simulink model "Neutral_current_Load_balancing"  (R2019b)
settings: Solver=ode3  StartTime=0.0  StopTime=1  FixedStep=1e-6  MaxStep=1e-5  RelTol=1e-3
libraries: powerlib x39, powerlib_meascontrol x12, simulink x3, dsparch4 x1, eeHysteresisControl x1
settings Model: Creator=ASUS  LastModifiedBy=ASUS

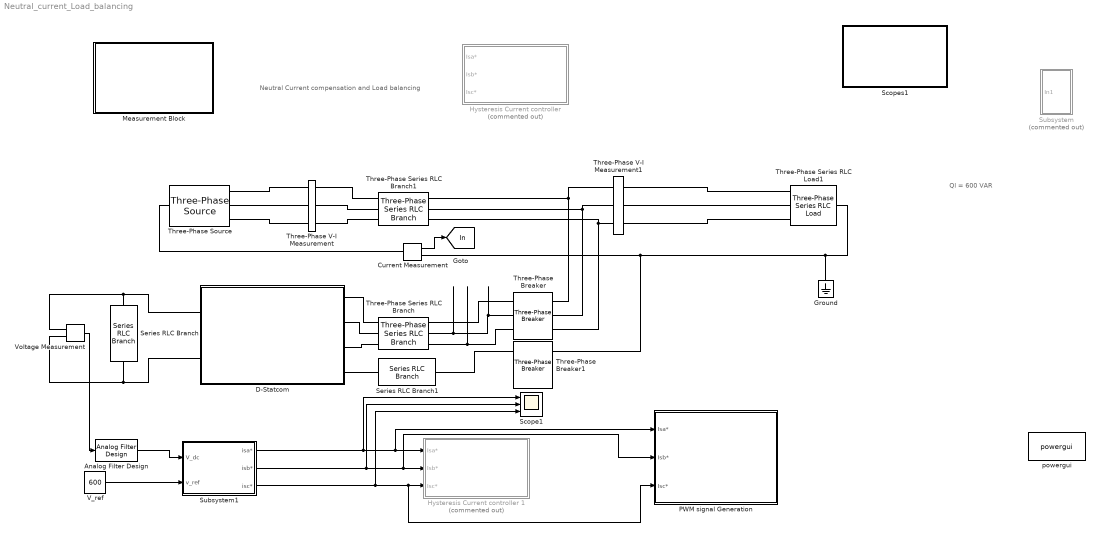
== system Neutral_current_Load_balancing ==
  note: Neutral Current compensation and Load balancing
  note: Ql = 600 VAR
  Analog Filter Design : dsparch4/Analog Filter Design  method=Butterworth  filttype=Lowpass  N=8  Wlo=75*2*pi  Whi=80  Rp=2  Rs=40
  Current Measurement : powerlib/Measurements/Current Measurement  PhasorSimulation=off  OutputType=Complex  PSBequivalent=0
      settings: SourceProductName=Simscape Electrical
  "D-Statcom " : Subsystem
  Ground : powerlib/Elements/Ground  LConnTagsString=a
      settings: SourceProductName=Simscape Electrical
  "Hysteresis Current controller " : Subsystem  Commented=on
  Hysteresis Current controller 1 : Subsystem  Commented=on
  Measurement Block : Subsystem
  PWM signal Generation : Subsystem
  Scope1 : Scope  NumInputPorts=3
  Scopes1 : Subsystem
  Series RLC Branch : powerlib/Elements/Series RLC Branch  LConnTagsString=__new0  RConnTagsString=__new0  BranchType=C  Resistance=1  Inductance=1e-3  SetiL0=off  InitialCurrent=0  Capacitance=10000e-6  Setx0=on  InitialVoltage=600  Measurements=None
      settings: SourceProductName=Simscape Electrical
  Series RLC Branch1 : powerlib/Elements/Series RLC Branch  LConnTagsString=__new0  RConnTagsString=__new0  BranchType=RL  Resistance=0.01  Inductance=12e-3  SetiL0=off  InitialCurrent=0  Capacitance=1e-6  Setx0=off  InitialVoltage=0  Measurements=None
      settings: SourceProductName=Simscape Electrical
  Subsystem : Subsystem  Commented=on
  Subsystem1 : Subsystem
  Three-Phase Series RLC Branch : powerlib/Elements/Three-Phase Series RLC Branch  LConnTagsString=A|B|C  RConnTagsString=A|B|C  BranchType=RL  Resistance=0.01  Inductance=10e-3  Capacitance=1e-6  Measurements=None
      settings: SourceProductName=Simscape Electrical
  Three-Phase Series RLC Branch1 : powerlib/Elements/Three-Phase Series RLC Branch  LConnTagsString=A|B|C  RConnTagsString=A|B|C  BranchType=RL  Resistance=0.01  Inductance=3.35e-3  Capacitance=1e-6  Measurements=None
      settings: SourceProductName=Simscape Electrical
  Three-Phase Series RLC Load1 : powerlib/Elements/Three-Phase Series RLC Load  LConnTagsString=A|B|C  RConnTagsString=N  Configuration=Y (neutral)  NominalVoltage=sqrt(6)*100  Vabc=[100 100 100]  Vabcp=[1e3 1e3 1e3]  NominalFrequency=50  UnbalancedPower=on  ActivePower=800  InductivePower=1000  CapacitivePower=0  Pabc=[100 200 300]  QLabc=[200 150 300]  QCabc=[0 0 0]  Pabcp=[10e3 9e3 11e3]  QLabcp=[100 90 110]  QCabcp=[100 90 110]  Measurements=None  LoadType=constant Z
      settings: SourceProductName=Simscape Electrical
  Three-Phase V-I Measurement : powerlib/Measurements/Three-Phase V-I Measurement  VoltageMeasurement=phase-to-ground  SetLabelV=on  LabelV=Vs  Vpu=off  VpuLL=off  CurrentMeasurement=yes  SetLabelI=on  LabelI=Is  Ipu=off  Pbase=100e6  Vbase=500e3  OutputType=Complex  PhasorSimulation=off  PSBequivalent=0
      settings: SourceProductName=Simscape Electrical
  Three-Phase V-I Measurement1 : powerlib/Measurements/Three-Phase V-I Measurement  VoltageMeasurement=phase-to-ground  SetLabelV=on  LabelV=Vr  Vpu=off  VpuLL=off  CurrentMeasurement=yes  SetLabelI=on  LabelI=Ir  Ipu=off  Pbase=100e6  Vbase=500e3  OutputType=Complex  PhasorSimulation=off  PSBequivalent=0
      settings: SourceProductName=Simscape Electrical
  Three-Phase Breaker : powerlib/Elements/Three-Phase Breaker  InitialState=open  SwitchA=on  SwitchB=on  SwitchC=on  SwitchTimes=[0.1 0.6]  External=off  BreakerResistance=0.01  SnubberResistance=1e6  SnubberCapacitance=inf  Measurements=None
      settings: SourceProductName=Simscape Electrical
  Three-Phase Breaker1 : powerlib/Elements/Three-Phase Breaker  InitialState=open  SwitchA=on  SwitchB=off  SwitchC=off  SwitchTimes=[0.1 0.6]  External=off  BreakerResistance=0.01  SnubberResistance=1e6  SnubberCapacitance=inf  Measurements=None
      settings: SourceProductName=Simscape Electrical
  Three-Phase Source : powerlib/Electrical Sources/Three-Phase Source  InternalConnection=Yn  VoltagePhases=off  Voltage=100*sqrt(6)  PhaseAngle=0  Voltage_phases=[25e3 25e3 25e3]/sqrt(3)  PhaseAngles_phases=[0 -120 +120]  Frequency=50  NonIdealSource=off  SpecifyImpedance=off  Resistance=0.8929  Inductance=16.58e-3  ShortCircuitLevel=100e6  BaseVoltage=sqrt(2)*100  XRratio=7  BusType=swing  Pref=10e3  Qref=0  Prefabc=[10e3, 10e3, 10e3]  Qrefabc=[0, 0, 0]  Qmin=-inf  Qmax=inf
      settings: SourceProductName=Simscape Electrical
  V_ref : Constant  Value=600
  Voltage Measurement : powerlib/Measurements/Voltage Measurement  PhasorSimulation=off  OutputType=Complex  PSBequivalent=0
      settings: SourceProductName=Simscape Electrical
  powergui : powerlib/powergui  Priority=1  SimulationMode=Discrete  SampleTime=1e-6  frequency=60  Iterations=50  frequencyindice=50  Pbase=100e6  ErrMax=1e-4  UnitsV=kV  UnitsW=MW  buscounter=0  FunctionMessages=off  echomessages=off  EnableUseOfTLC=off  CurrentSourceSwitches=off  DisableSnubberDevices=off  DisableRonSwitches=off  DisableVfSwitches=off  DisplayEquations=off  AutomaticDiscreteSolvers=off  SolverType=Tustin/Backward Euler (TBE)  Interpol=off  ExternalGateDelay=off  methode=off  Ts=100  x0status=blocks  SPID=on  SwTol=0  HookPort=off  NonlinearTolerance=1e-4  nMaxIteration=100  ContinueOnMaxIteration=off  RestoreLinks=warning  ResistiveCurrentMeasurement=off  Frange=[0:2:500]  Ylog=off  Xlog=on  ShowGrid=off  save=off  variable=ZData  structure=0  ZoomFFT=off  StartTime=0.0  cycles=1  DisplayStyle=1  fundamental=60  FreqAxis=off  MaxFrequency=1000  frequencyindicesteady=1  RmsSteady=1  display=off
      settings: SourceProductName=Simscape Electrical
  tag scope: In=global
  wires:
  Subsystem1/1(isa*) -> PWM signal Generation/1(Isa*), Hysteresis Current controller 1/1(Isa*), Scope1/1
  Subsystem1/2(isb*) -> PWM signal Generation/2(Isb*), Hysteresis Current controller 1/2(Isb*), Scope1/2
  Subsystem1/3(isc*) -> PWM signal Generation/3(Isc*), Hysteresis Current controller 1/3(Isc*), Scope1/3
  V_ref/1 -> Subsystem1/2(v_ref)
  Voltage Measurement/1 -> Analog Filter Design/1
  Analog Filter Design/1 -> Subsystem1/1(V_dc)
  Current Measurement/1 -> [In]
  connections:
  Three-Phase Series RLC Branch/LConn1 -- "D-Statcom "/RConn1
  "D-Statcom "/RConn2 -- Three-Phase Series RLC Branch/LConn2
  "D-Statcom "/RConn3 -- Three-Phase Series RLC Branch/LConn3
  "D-Statcom "/LConn1 -- Voltage Measurement/LConn1 -- Series RLC Branch/LConn1
  "D-Statcom "/LConn2 -- Series RLC Branch/RConn1 -- Voltage Measurement/LConn2
  Three-Phase V-I Measurement/LConn1 -- Three-Phase Source/RConn1
  Three-Phase Source/RConn2 -- Three-Phase V-I Measurement/LConn2
  Three-Phase Source/RConn3 -- Three-Phase V-I Measurement/LConn3
  Three-Phase Breaker/RConn1 -- Three-Phase V-I Measurement1/LConn1 -- Three-Phase Series RLC Branch1/RConn1
  Three-Phase Breaker/RConn2 -- Three-Phase V-I Measurement1/LConn2 -- Three-Phase Series RLC Branch1/RConn2
  Three-Phase Breaker/RConn3 -- Three-Phase Series RLC Branch1/RConn3 -- Three-Phase V-I Measurement1/LConn3
  Three-Phase Series RLC Load1/LConn1 -- Three-Phase V-I Measurement1/RConn1
  Three-Phase Series RLC Load1/LConn2 -- Three-Phase V-I Measurement1/RConn2
  Three-Phase Series RLC Load1/LConn3 -- Three-Phase V-I Measurement1/RConn3
  Three-Phase Breaker/LConn1 -- Three-Phase Series RLC Branch/RConn1
  Three-Phase Breaker/LConn2 -- Three-Phase Series RLC Branch/RConn2
  Three-Phase Breaker/LConn3 -- Three-Phase Series RLC Branch/RConn3
  Three-Phase Series RLC Branch1/LConn1 -- Three-Phase V-I Measurement/RConn1
  Three-Phase V-I Measurement/RConn2 -- Three-Phase Series RLC Branch1/LConn2
  Three-Phase Series RLC Branch1/LConn3 -- Three-Phase V-I Measurement/RConn3
  Series RLC Branch1/LConn1 -- "D-Statcom "/RConn4
  Current Measurement/RConn1 -- Three-Phase Breaker1/RConn1 -- Ground/LConn1 -- Three-Phase Series RLC Load1/RConn1
  Series RLC Branch1/RConn1 -- Three-Phase Breaker1/LConn1
  Current Measurement/LConn1 -- Three-Phase Source/LConn1

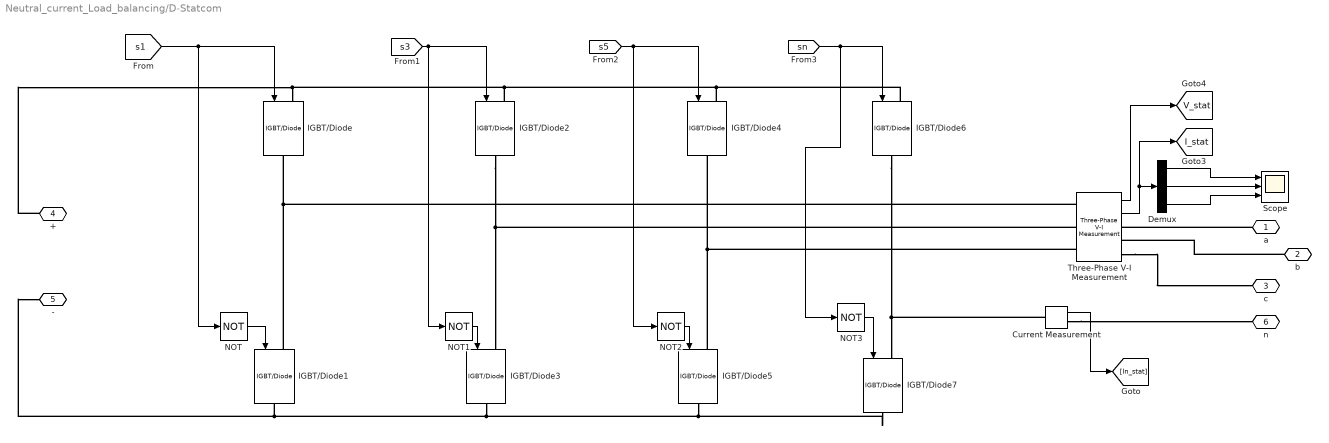
== system Neutral_current_Load_balancing/D-Statcom  ==
  Current Measurement : powerlib/Measurements/Current Measurement  PhasorSimulation=off  OutputType=Complex  PSBequivalent=0
      settings: SourceProductName=Simscape Electrical
  Demux : Demux  Outputs=3
  IGBT/Diode{,1..7} (8 alike) : powerlib/Power Electronics/IGBT//Diode  Ron=1e-3  Rs=1e5  Cs=inf  Measurements=off
      settings: SourceProductName=Simscape Electrical
  NOT{,1..3} (4 alike) : Logic  Operator=NOT  IconShape=distinctive  AllPortsSameDT=off  OutDataTypeStr=boolean
  Scope : Scope  NumInputPorts=3
  Three-Phase V-I Measurement : powerlib/Measurements/Three-Phase V-I Measurement  VoltageMeasurement=phase-to-ground  SetLabelV=off  LabelV=Vabc  Vpu=off  VpuLL=off  CurrentMeasurement=yes  SetLabelI=off  LabelI=Iabc  Ipu=off  Pbase=100e6  Vbase=500e3  OutputType=Complex  PhasorSimulation=off  PSBequivalent=0
      settings: SourceProductName=Simscape Electrical
  a : PMIOPort  Side=Right
  b : PMIOPort  Port=2  Side=Right
  c : PMIOPort  Port=3  Side=Right
  + : PMIOPort  Port=4  Side=Left
  - : PMIOPort  Port=5  Side=Left
  n : PMIOPort  Port=6  Side=Right
  tag scope: I_stat=global, V_stat=global
  wires:
  [s1] -> NOT/1, IGBT/Diode/1
  [s5] -> NOT2/1, IGBT/Diode4/1
  NOT2/1 -> IGBT/Diode5/1
  NOT/1 -> IGBT/Diode1/1
  [s3] -> IGBT/Diode2/1, NOT1/1
  NOT1/1 -> IGBT/Diode3/1
  Three-Phase V-I Measurement/2 -> [I_stat], Demux/1
  Demux/1 -> Scope/1
  Demux/2 -> Scope/2
  Demux/3 -> Scope/3
  Three-Phase V-I Measurement/1 -> [V_stat]
  [sn] -> NOT3/1, IGBT/Diode6/1
  NOT3/1 -> IGBT/Diode7/1
  Current Measurement/1 -> [In_stat]
  connections:
  IGBT/Diode1/RConn1 -- -/RConn1 -- IGBT/Diode7/RConn1 -- IGBT/Diode5/RConn1 -- IGBT/Diode3/RConn1
  IGBT/Diode2/LConn1 -- IGBT/Diode6/LConn1 -- IGBT/Diode4/LConn1 -- +/RConn1 -- IGBT/Diode/LConn1
  IGBT/Diode1/LConn1 -- Three-Phase V-I Measurement/LConn1 -- IGBT/Diode/RConn1
  IGBT/Diode2/RConn1 -- IGBT/Diode3/LConn1 -- Three-Phase V-I Measurement/LConn2
  IGBT/Diode5/LConn1 -- Three-Phase V-I Measurement/LConn3 -- IGBT/Diode4/RConn1
  a/RConn1 -- Three-Phase V-I Measurement/RConn1
  b/RConn1 -- Three-Phase V-I Measurement/RConn2
  Three-Phase V-I Measurement/RConn3 -- c/RConn1
  IGBT/Diode6/RConn1 -- Current Measurement/LConn1 -- IGBT/Diode7/LConn1
  Current Measurement/RConn1 -- n/RConn1

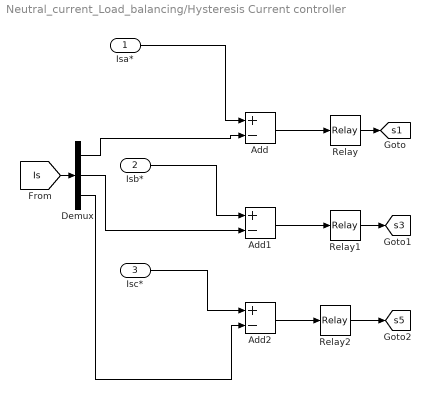
== system Neutral_current_Load_balancing/Hysteresis Current controller  ==
  Isa* : Inport
  Isb* : Inport  Port=2
  Isc* : Inport  Port=3
  Add : Sum  Inputs=+-
  Add1 : Sum  Inputs=+-
  Add2 : Sum  Inputs=+-
  Demux : Demux  Outputs=3
  Relay : Relay  OnSwitchValue=0.1  OffSwitchValue=-0.1
  Relay1 : Relay  OnSwitchValue=0.1  OffSwitchValue=-0.1
  Relay2 : Relay  OnSwitchValue=0.1  OffSwitchValue=-0.1
  tag scope: s1=global, s3=global, s5=global
  wires:
  Add1/1 -> Relay1/1
  Relay2/1 -> [s5]
  Add/1 -> Relay/1
  Add2/1 -> Relay2/1
  Relay/1 -> [s1]
  Isa*/1 -> Add/1
  Isc*/1 -> Add2/1
  Relay1/1 -> [s3]
  Isb*/1 -> Add1/1
  Demux/2 -> Add1/2
  [Is] -> Demux/1
  Demux/3 -> Add2/2
  Demux/1 -> Add/2

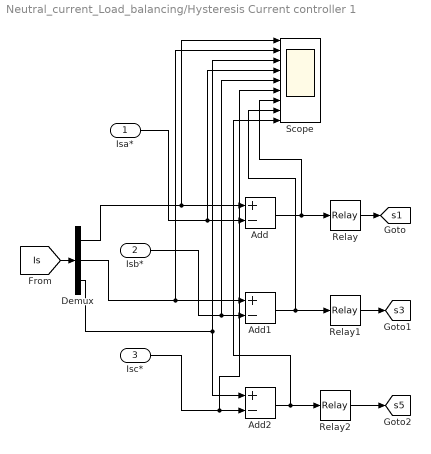
== system Neutral_current_Load_balancing/Hysteresis Current controller 1 ==
  Isa* : Inport
  Isb* : Inport  Port=2
  Isc* : Inport  Port=3
  Add : Sum  Inputs=+-
  Add1 : Sum  Inputs=+-
  Add2 : Sum  Inputs=+-
  Demux : Demux  Outputs=3
  Relay : Relay  OnSwitchValue=0.01  OffSwitchValue=-0.01
  Relay1 : Relay  OnSwitchValue=0.01  OffSwitchValue=-0.01
  Relay2 : Relay  OnSwitchValue=0.01  OffSwitchValue=-0.01
  Scope : Scope  NumInputPorts=9
  tag scope: s1=global, s3=global, s5=global
  wires:
  Add1/1 -> Scope/8, Relay1/1
  Relay2/1 -> [s5]
  Add/1 -> Scope/7, Relay/1
  Add2/1 -> Scope/9, Relay2/1
  Relay/1 -> [s1]
  Isa*/1 -> Scope/4, Add/2
  Isc*/1 -> Scope/6, Add2/2
  Relay1/1 -> [s3]
  Isb*/1 -> Scope/5, Add1/2
  Demux/2 -> Scope/2, Add1/1
  [Is] -> Demux/1
  Demux/3 -> Scope/3, Add2/1
  Demux/1 -> Scope/1, Add/1

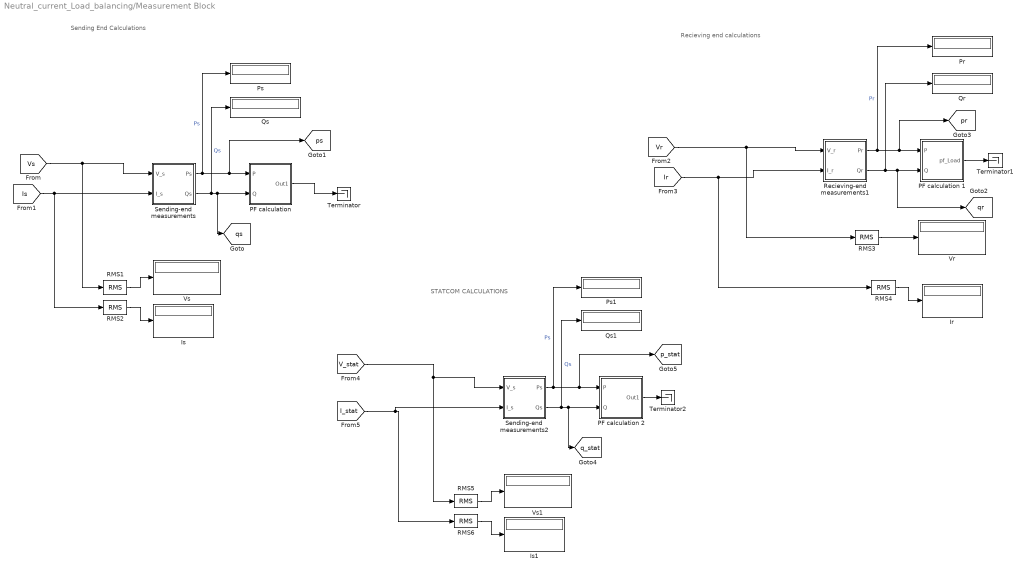
== system Neutral_current_Load_balancing/Measurement Block ==
  note: STATCOM CALCULATIONS
  note: Recieving end calculations
  note: Sending End Calculations
  Ir : Display
  Is : Display
  Is1 : Display
  "PF calculation " : Subsystem
  PF calculation 1 : Subsystem
  PF calculation 2 : Subsystem
  Pr : Display
  Ps : Display
  Ps1 : Display
  Qr : Display
  Qs : Display
      settings: Format=short_e
  Qs1 : Display
  RMS{1..6} (6 alike) : powerlib_meascontrol/Measurements/RMS  TrueRMS=on  Freq=60  RMSInit=120  Ts=0
      settings: SourceProductName=Simscape Electrical
  Recieving-end measurements1 : Subsystem
  Sending-end measurements : Subsystem
  Sending-end measurements2 : Subsystem
  Terminator : Terminator
  Terminator1 : Terminator
  Terminator2 : Terminator
  Vr : Display
  Vs : Display
  Vs1 : Display
  tag scope: p_stat=global, pr=global, ps=global, q_stat=global, qr=global, qs=global
  wires:
  Sending-end measurements/1(Ps) -> Ps/1, [ps], "PF calculation "/1(P)  "Ps"
  Sending-end measurements/2(Qs) -> Qs/1, [qs], "PF calculation "/2(Q)  "Qs"
  [Is] -> RMS2/1, Sending-end measurements/2(I_s)
  Recieving-end measurements1/2(Qr) -> Qr/1, [qr], PF calculation 1/2(Q)
  Recieving-end measurements1/1(Pr) -> Pr/1, [pr], PF calculation 1/1(P)  "Pr"
  RMS1/1 -> Vs/1
  RMS2/1 -> Is/1
  [Vs] -> Sending-end measurements/1(V_s), RMS1/1
  RMS3/1 -> Vr/1
  [Vr] -> RMS3/1, Recieving-end measurements1/1(V_r)
  RMS4/1 -> Ir/1
  [Ir] -> RMS4/1, Recieving-end measurements1/2(I_r)
  Sending-end measurements2/2(Qs) -> Qs1/1, [q_stat], PF calculation 2/2(Q)  "Qs"
  Sending-end measurements2/1(Ps) -> Ps1/1, [p_stat], PF calculation 2/1(P)  "Ps"
  [V_stat] -> Sending-end measurements2/1(V_s), RMS5/1
  RMS5/1 -> Vs1/1
  RMS6/1 -> Is1/1
  [I_stat] -> Sending-end measurements2/2(I_s), RMS6/1
  "PF calculation "/1(Out1) -> Terminator/1
  PF calculation 1/1(pf_Load) -> Terminator1/1
  PF calculation 2/1(Out1) -> Terminator2/1

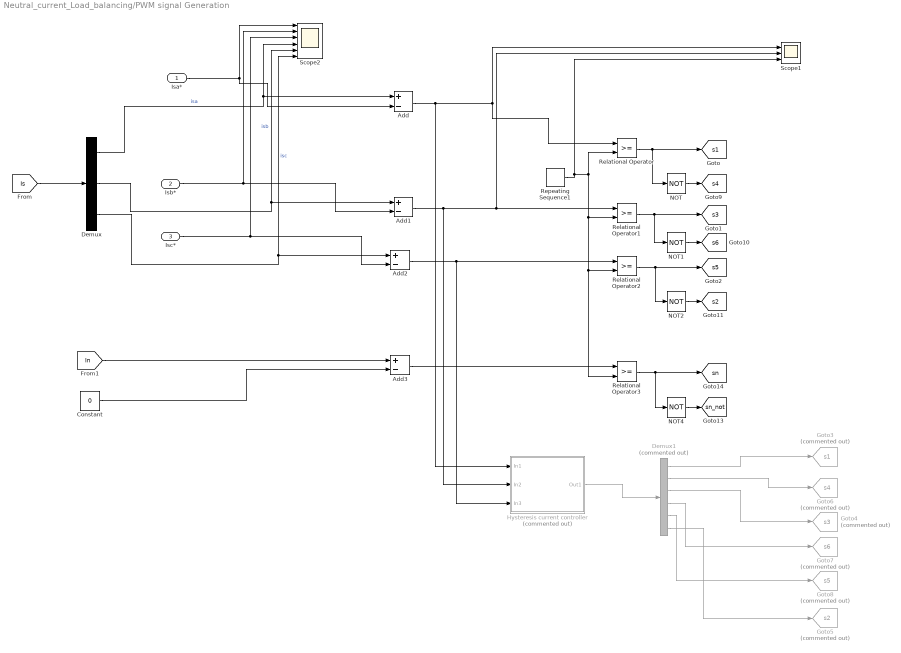
== system Neutral_current_Load_balancing/PWM signal Generation ==
  Isa* : Inport
  Isb* : Inport  Port=2
  Isc* : Inport  Port=3
  Add{,1..3} (4 alike) : Sum  Inputs=+-
  Constant : Constant  Value=0
  Demux : Demux  Outputs=3
  Demux1 : Demux  Commented=on  Outputs=6
  Goto3 : Goto  Commented=on  GotoTag=s1  TagVisibility=global
  Goto4 : Goto  Commented=on  GotoTag=s3  TagVisibility=global
  Goto5 : Goto  Commented=on  GotoTag=s2  TagVisibility=global
  Goto6 : Goto  Commented=on  GotoTag=s4  TagVisibility=global
  Goto7 : Goto  Commented=on  GotoTag=s6  TagVisibility=global
  Goto8 : Goto  Commented=on  GotoTag=s5  TagVisibility=global
  Hysteresis current controller : Subsystem  Commented=on
  NOT{,1..2,4} (4 alike) : Logic  Operator=NOT  IconShape=distinctive  AllPortsSameDT=off  OutDataTypeStr=boolean
  Relational Operator{,1..3} (4 alike) : RelationalOperator  OutDataTypeStr=boolean  RndMeth=Simplest
  Repeating Sequence1 : simulink/Sources/Repeating Sequence  rep_seq_t=[0 1/4 1/2 3/4 1]*1/20000  rep_seq_y=[0 2 0 -2 0]
  Scope1 : Scope  NumInputPorts=3
  Scope2 : Scope  NumInputPorts=6
  tag scope: s1=global, s2=global, s3=global, s4=global, s5=global, s6=global, sn=global, sn_not=global
  wires:
  Relational Operator1/1 -> NOT1/1, [s3]
  Relational Operator2/1 -> NOT2/1, [s5]
  Relational Operator/1 -> NOT/1, [s1]
  Isc*/1 -> Add2/2, Scope2/3
  Isa*/1 -> Add/2, Scope2/1
  Isb*/1 -> Add1/2, Scope2/2
  Demux/3 -> Add2/1, Scope2/6  "isc"
  [Is] -> Demux/1
  Demux/1 -> Add/1, Scope2/4  "isa"
  Demux/2 -> Add1/1, Scope2/5  "isb"
  Demux1/1 -> Goto3/1
  Demux1/2 -> Goto6/1
  Demux1/3 -> Goto4/1
  Demux1/4 -> Goto7/1
  Demux1/5 -> Goto8/1
  Demux1/6 -> Goto5/1
  Hysteresis current controller/1(Out1) -> Demux1/1
  NOT/1 -> [s4]
  NOT1/1 -> [s6]
  NOT2/1 -> [s2]
  Add/1 -> Relational Operator/1, Scope1/1, Hysteresis current controller/1(In1)
  Add1/1 -> Scope1/2, Relational Operator1/1, Hysteresis current controller/2(In2)
  Add2/1 -> Relational Operator2/1, Hysteresis current controller/3(In3)
  Add3/1 -> Relational Operator3/1
  NOT4/1 -> [sn_not]
  Repeating Sequence1/1 -> Scope1/3, Relational Operator3/2, Relational Operator2/2, Relational Operator1/2, Relational Operator/2
  Relational Operator3/1 -> [sn], NOT4/1
  [In] -> Add3/1
  Constant/1 -> Add3/2

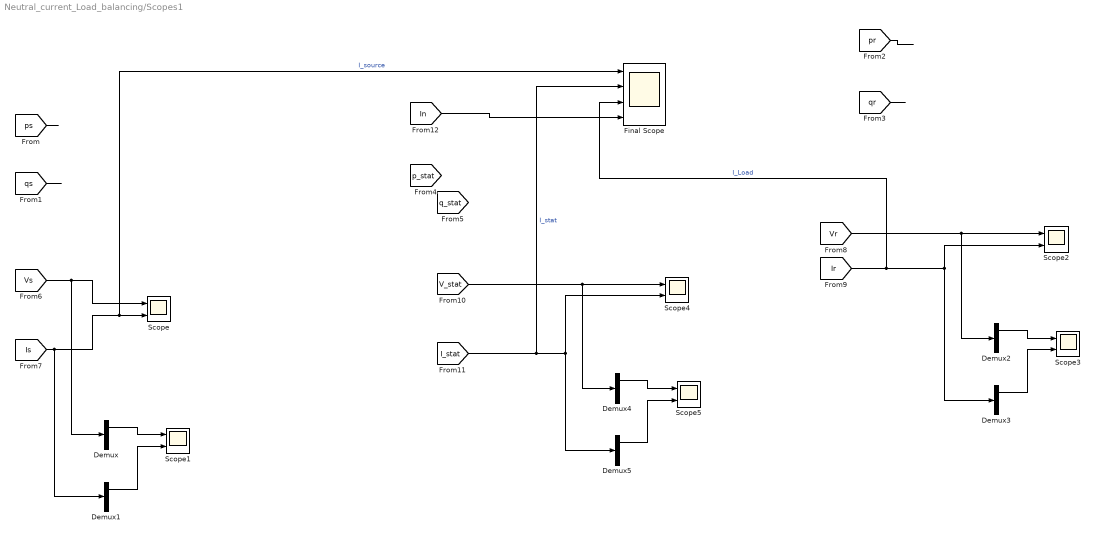
== system Neutral_current_Load_balancing/Scopes1 ==
  Demux{,1..5} (6 alike) : Demux  Outputs=3
  Final Scope : Scope  NumInputPorts=4
  Scope{,1..5} (6 alike) : Scope  NumInputPorts=2
  wires:
  [ps] -> ?
  [qr] -> ?
  [pr] -> ?
  [qs] -> ?
  [Vs] -> Demux/1, Scope/1
  [Is] -> Demux1/1, Final Scope/1, Scope/2  "I_source"
  Demux/1 -> Scope1/1
  Demux1/1 -> Scope1/2
  Demux3/1 -> Scope3/2
  Demux2/1 -> Scope3/1
  [Ir] -> Final Scope/3, Demux3/1, Scope2/2  "I_Load"
  [Vr] -> Demux2/1, Scope2/1
  [V_stat] -> Scope4/1, Demux4/1
  [I_stat] -> Final Scope/2, Scope4/2, Demux5/1  "I_stat"
  Demux4/1 -> Scope5/1
  Demux5/1 -> Scope5/2
  [In] -> Final Scope/4

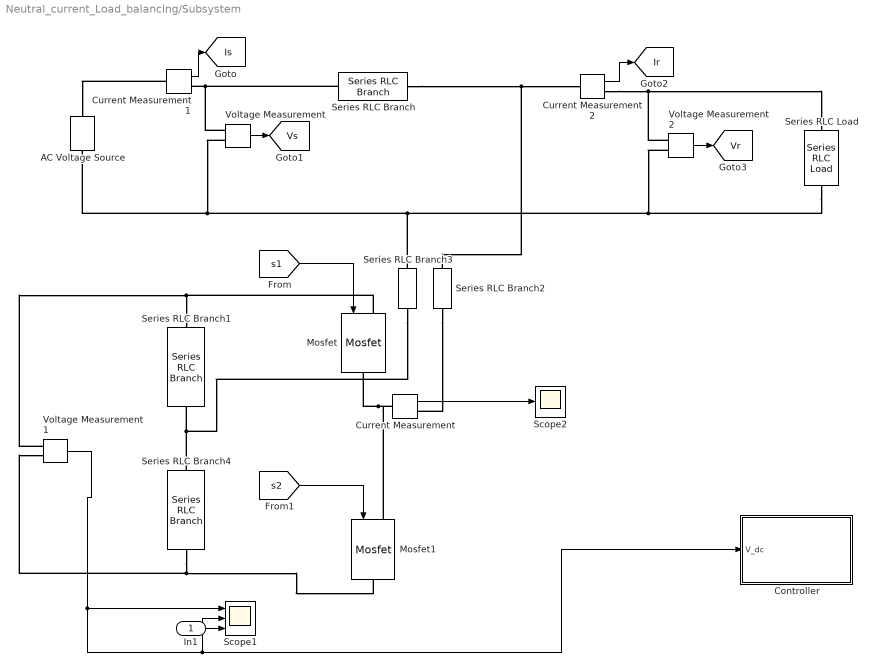
== system Neutral_current_Load_balancing/Subsystem ==
  In1 : Inport
  AC Voltage Source : powerlib/Electrical Sources/AC Voltage Source  Amplitude=311  Phase=0  Frequency=50  SampleTime=0  Measurements=None  BusType=swing  Pref=10e3  Qref=0  Qmin=-inf  Qmax=+inf
      settings: SourceProductName=Simscape Electrical
  Controller : Subsystem
  Current Measurement : powerlib/Measurements/Current Measurement  PhasorSimulation=off  OutputType=Complex  PSBequivalent=0
      settings: SourceProductName=Simscape Electrical
  Current Measurement1 : powerlib/Measurements/Current Measurement  PhasorSimulation=off  OutputType=Complex  PSBequivalent=0
      settings: SourceProductName=Simscape Electrical
  Current Measurement2 : powerlib/Measurements/Current Measurement  PhasorSimulation=off  OutputType=Complex  PSBequivalent=0
      settings: SourceProductName=Simscape Electrical
  Mosfet : powerlib/Power Electronics/Mosfet  Ron=0.01  Lon=0  Rd=0.01  Vfd=0  IC=0  Rs=1e5  Cs=inf  Measurements=off
      settings: SourceProductName=Simscape Electrical
  Mosfet1 : powerlib/Power Electronics/Mosfet  Ron=0.01  Lon=0  Rd=0.01  Vfd=0  IC=0  Rs=1e5  Cs=inf  Measurements=off
      settings: SourceProductName=Simscape Electrical
  Scope1 : Scope  NumInputPorts=3
  Scope2 : Scope
  Series RLC Branch : powerlib/Elements/Series RLC Branch  LConnTagsString=__new0  RConnTagsString=__new0  BranchType=R  Resistance=0.01  Inductance=1e-3  SetiL0=off  InitialCurrent=0  Capacitance=1e-6  Setx0=off  InitialVoltage=0  Measurements=None
      settings: SourceProductName=Simscape Electrical
  Series RLC Branch1 : powerlib/Elements/Series RLC Branch  LConnTagsString=__new0  RConnTagsString=__new0  BranchType=C  Resistance=1  Inductance=1e-3  SetiL0=off  InitialCurrent=0  Capacitance=10000e-6  Setx0=off  InitialVoltage=0  Measurements=None
      settings: SourceProductName=Simscape Electrical
  Series RLC Branch2 : powerlib/Elements/Series RLC Branch  LConnTagsString=__new0  RConnTagsString=__new0  BranchType=L  Resistance=1  Inductance=0.06  SetiL0=off  InitialCurrent=0  Capacitance=1e-6  Setx0=off  InitialVoltage=0  Measurements=None
      settings: SourceProductName=Simscape Electrical
  Series RLC Branch3 : powerlib/Elements/Series RLC Branch  LConnTagsString=__new0  RConnTagsString=__new0  BranchType=L  Resistance=1  Inductance=0.06  SetiL0=off  InitialCurrent=0  Capacitance=1e-6  Setx0=off  InitialVoltage=0  Measurements=None
      settings: SourceProductName=Simscape Electrical
  Series RLC Branch4 : powerlib/Elements/Series RLC Branch  LConnTagsString=__new0  RConnTagsString=__new0  BranchType=C  Resistance=1  Inductance=1e-3  SetiL0=off  InitialCurrent=0  Capacitance=10000e-6  Setx0=off  InitialVoltage=0  Measurements=None
      settings: SourceProductName=Simscape Electrical
  Series RLC Load : powerlib/Elements/Series RLC Load  LConnTagsString=a  RConnTagsString=__new0  NominalVoltage=222  NominalFrequency=50  ActivePower=300  InductivePower=500  CapacitivePower=0  Setx0=off  InitialVoltage=0  SetiL0=off  InitialCurrent=0  Measurements=None  LoadType=constant Z
      settings: SourceProductName=Simscape Electrical
  Voltage Measurement : powerlib/Measurements/Voltage Measurement  PhasorSimulation=off  OutputType=Complex  PSBequivalent=0
      settings: SourceProductName=Simscape Electrical
  Voltage Measurement1 : powerlib/Measurements/Voltage Measurement  PhasorSimulation=off  OutputType=Complex  PSBequivalent=0
      settings: SourceProductName=Simscape Electrical
  Voltage Measurement2 : powerlib/Measurements/Voltage Measurement  PhasorSimulation=off  OutputType=Complex  PSBequivalent=0
      settings: SourceProductName=Simscape Electrical
  tag scope: Ir=global, Is=global, Vr=global, Vs=global
  wires:
  Voltage Measurement1/1 -> Scope1/2, Controller/1(V_dc), Scope1/1
  Voltage Measurement/1 -> [Vs]
  Current Measurement/1 -> Scope2/1
  [s1] -> Mosfet/1
  Current Measurement1/1 -> [Is]
  Current Measurement2/1 -> [Ir]
  In1/1 -> Scope1/3
  [s2] -> Mosfet1/1
  Voltage Measurement2/1 -> [Vr]
  connections:
  Current Measurement2/RConn1 -- Voltage Measurement2/LConn1 -- Series RLC Load/LConn1
  Voltage Measurement/LConn2 -- Series RLC Load/RConn1 -- Voltage Measurement2/LConn2 -- Series RLC Branch3/LConn1 -- AC Voltage Source/LConn1
  Series RLC Branch/RConn1 -- Series RLC Branch2/LConn1 -- Current Measurement2/LConn1
  Series RLC Branch4/LConn1 -- Series RLC Branch3/RConn1 -- Series RLC Branch1/RConn1
  Voltage Measurement1/LConn1 -- Mosfet/LConn1 -- Series RLC Branch1/LConn1
  Current Measurement/LConn1 -- Mosfet/RConn1 -- Mosfet1/LConn1
  Series RLC Branch4/RConn1 -- Mosfet1/RConn1 -- Voltage Measurement1/LConn2
  Series RLC Branch2/RConn1 -- Current Measurement/RConn1
  Series RLC Branch/LConn1 -- Voltage Measurement/LConn1 -- Current Measurement1/RConn1
  Current Measurement1/LConn1 -- AC Voltage Source/RConn1

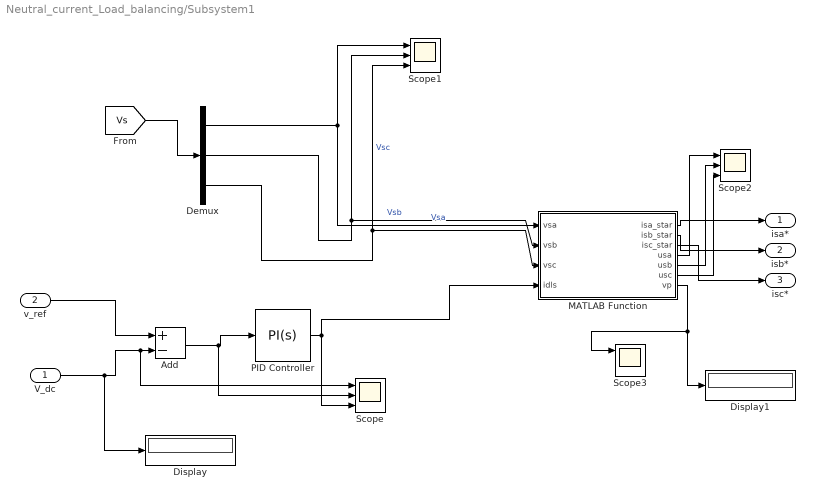
== system Neutral_current_Load_balancing/Subsystem1 ==
  V_dc : Inport
  v_ref : Inport  Port=2
  Add : Sum  Inputs=+-
  Demux : Demux  Outputs=3
  Display : Display
  Display1 : Display
  MATLAB Function : MATLAB Function  TreatAsAtomicUnit=on
  PID Controller : simulink/Continuous/PID Controller  Controller=PI  Form=Parallel  TimeDomain=Continuous-time  SampleTime=1e-6  IntegratorMethod=Forward Euler  FilterMethod=Forward Euler  ControllerParametersSource=internal  P=0.3  I=0.903  D=0  UseFilter=on  N=100  TunerSelectOption=Transfer Function Based (PID Tuner App)  ZeroCross=off  InitialConditionSource=internal  InitialConditionForIntegrator=0  InitialConditionForFilter=0  DifferentiatorICPrevScaledInput=0  ExternalReset=none  TrackingMode=off  Kt=1  LimitOutput=off  UpperSaturationLimit=300  LowerSaturationLimit=-300  LinearizeAsGain=on  AntiWindupMode=none  Kb=1  RndMeth=Ceiling  POutMin=[]  POutMax=[]  IOutMin=[]  IOutMax=[]  DOutMin=[]  DOutMax=[]  NOutMin=[]  NOutMax=[]  SumOutMin=[]  SumOutMax=[]  SaturationOutMin=[]  SaturationOutMax=[]  PParamMin=[]  PParamMax=[]  IParamMin=[]  IParamMax=[]  DParamMin=[]  DParamMax=[]  NParamMin=[]  NParamMax=[]  KbParamMin=[]  KbParamMax=[]  KtParamMin=[]  KtParamMax=[]  KbOutMin=[]  KbOutMax=[]  KtOutMin=[]  KtOutMax=[]  IntegratorOutMin=[]  IntegratorOutMax=[]  FilterOutMin=[]  FilterOutMax=[]  SumI1OutMin=[]  SumI1OutMax=[]  SumI2OutMin=[]  SumI2OutMax=[]  SumI3OutMin=[]  SumI3OutMax=[]  SumI4OutMin=[]  SumI4OutMax=[]  SumDOutMin=[]  SumDOutMax=[]  DifferentiatorOutMin=[]  DifferentiatorOutMax=[]  FilterDiffOutCoefMin=[]  FilterDiffOutCoefMax=[]  ReciprocalOutMin=[]  ReciprocalOutMax=[]  SumDenOutMin=[]  SumDenOutMax=[]  SumNumOutMin=[]  SumNumOutMax=[]  DivideOutMin=[]  DivideOutMax=[]  IntegratorContinuousStateAttributes=''  IntegratorStateMustResolveToSignalObject=off  IntegratorRTWStateStorageClass=Auto  FilterContinuousStateAttributes=''  FilterStateMustResolveToSignalObject=off  FilterRTWStateStorageClass=Auto  ParallelPVariant=InternalParameters  IdealPVariant=Disabled  IVariant=InternalParameters  DVariant=Disabled  IntegratorVariant=Continuous  SatVariant=Disabled  AWVariant=Passthrough  PCopyVariant=Disabled  TRVariant=Disabled  FdbkBlocksVariant=Forward  IdealPFdbkVariant=Disabled  SatFdbkVariant=Disabled  DerivativeFilterVariant=Disabled  NVariant=Disabled  NCopyVariant=Disabled_SignalSpec  FilterICVariant=Disabled  IntegratorICVariant=InternalICs  ExternalResetVariant=Disabled  TRSumVariant=Passthrough  SumFdbkVariant=Disabled  SumVariant=Sum_PI
  Scope{,1..3} (4 alike) : Scope  NumInputPorts=3
  isa* : Outport
  isb* : Outport  Port=2
  isc* : Outport  Port=3
  wires:
  PID Controller/1 -> Scope/3, MATLAB Function/4(idls)
  v_ref/1 -> Add/1
  Add/1 -> Scope/2, PID Controller/1
  Demux/3 -> Scope1/3, MATLAB Function/3(vsc)  "Vsc"
  [Vs] -> Demux/1
  Demux/1 -> Scope1/1, MATLAB Function/1(vsa)  "Vsa"
  Demux/2 -> Scope1/2, MATLAB Function/2(vsb)  "Vsb"
  MATLAB Function/1(isa_star) -> isa*/1
  MATLAB Function/2(isb_star) -> isb*/1
  MATLAB Function/3(isc_star) -> isc*/1
  V_dc/1 -> Display/1, Scope/1, Add/2
  MATLAB Function/7(vp) -> Scope3/1, Display1/1
  MATLAB Function/4(usa) -> Scope2/1
  MATLAB Function/5(usb) -> Scope2/2
  MATLAB Function/6(usc) -> Scope2/3

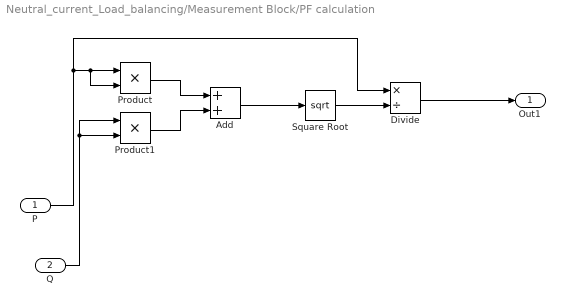
== system Neutral_current_Load_balancing/Measurement Block/PF calculation  ==
  P : Inport
  Q : Inport  Port=2
  Add : Sum
  Divide : Product  Inputs=*/
  Product : Product
  Product1 : Product
  Square Root : Sqrt  SaturateOnIntegerOverflow=on
  Out1 : Outport
  wires:
  Divide/1 -> Out1/1
  P/1 -> Divide/1, Product/2, Product/1
  Product/1 -> Add/1
  Add/1 -> Square Root/1
  Q/1 -> Product1/1, Product1/2
  Square Root/1 -> Divide/2
  Product1/1 -> Add/2

== system Neutral_current_Load_balancing/Measurement Block/PF calculation 1 ==
  P : Inport
  Q : Inport  Port=2
  Add : Sum
  Divide : Product  Inputs=*/
  Product : Product
  Product1 : Product
  Square Root : Sqrt  SaturateOnIntegerOverflow=on
  pf_Load : Outport
  wires:
  Divide/1 -> pf_Load/1
  P/1 -> Divide/1, Product/2, Product/1
  Product/1 -> Add/1
  Add/1 -> Square Root/1
  Q/1 -> Product1/1, Product1/2
  Square Root/1 -> Divide/2
  Product1/1 -> Add/2

== system Neutral_current_Load_balancing/Measurement Block/PF calculation 2 ==
  P : Inport
  Q : Inport  Port=2
  Add : Sum
  Divide : Product  Inputs=*/
  Product : Product
  Product1 : Product
  Square Root : Sqrt  SaturateOnIntegerOverflow=on
  Out1 : Outport
  wires:
  Divide/1 -> Out1/1
  P/1 -> Divide/1, Product/2, Product/1
  Product/1 -> Add/1
  Add/1 -> Square Root/1
  Q/1 -> Product1/1, Product1/2
  Square Root/1 -> Divide/2
  Product1/1 -> Add/2

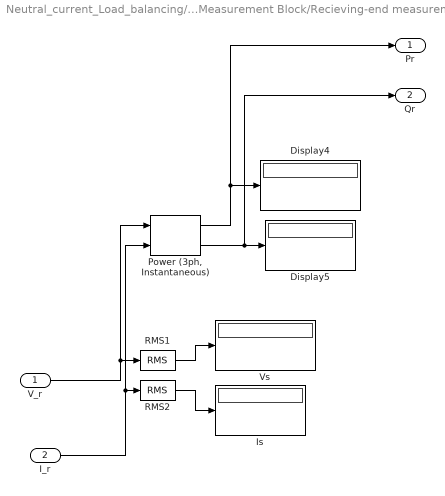
== system Neutral_current_Load_balancing/Measurement Block/Recieving-end measurements1 ==
  V_r : Inport
  I_r : Inport  Port=2
  Display4 : Display
  Display5 : Display
  Is : Display
  "Power (3ph, Instantaneous)" : powerlib_meascontrol/Measurements/Power (3ph, Instantaneous)
      settings: SourceProductName=Simscape Electrical
  RMS1 : powerlib_meascontrol/Measurements/RMS  TrueRMS=on  Freq=60  RMSInit=120  Ts=0
      settings: SourceProductName=Simscape Electrical
  RMS2 : powerlib_meascontrol/Measurements/RMS  TrueRMS=on  Freq=60  RMSInit=120  Ts=0
      settings: SourceProductName=Simscape Electrical
  Vs : Display
  Pr : Outport
  Qr : Outport  Port=2
  wires:
  RMS2/1 -> Is/1
  "Power (3ph, Instantaneous)"/1 -> Pr/1, Display4/1
  "Power (3ph, Instantaneous)"/2 -> Qr/1, Display5/1
  V_r/1 -> "Power (3ph, Instantaneous)"/1, RMS1/1
  I_r/1 -> "Power (3ph, Instantaneous)"/2, RMS2/1
  RMS1/1 -> Vs/1

== system Neutral_current_Load_balancing/Measurement Block/Sending-end measurements ==
  V_s : Inport
  I_s : Inport  Port=2
  "Power (3ph, Instantaneous)" : powerlib_meascontrol/Measurements/Power (3ph, Instantaneous)
      settings: SourceProductName=Simscape Electrical
  Ps : Outport
  Qs : Outport  Port=2
  wires:
  "Power (3ph, Instantaneous)"/1 -> Ps/1
  "Power (3ph, Instantaneous)"/2 -> Qs/1
  V_s/1 -> "Power (3ph, Instantaneous)"/1
  I_s/1 -> "Power (3ph, Instantaneous)"/2

== system Neutral_current_Load_balancing/Measurement Block/Sending-end measurements2 ==
  V_s : Inport
  I_s : Inport  Port=2
  "Power (3ph, Instantaneous)" : powerlib_meascontrol/Measurements/Power (3ph, Instantaneous)
      settings: SourceProductName=Simscape Electrical
  Ps : Outport
  Qs : Outport  Port=2
  wires:
  "Power (3ph, Instantaneous)"/1 -> Ps/1
  "Power (3ph, Instantaneous)"/2 -> Qs/1
  V_s/1 -> "Power (3ph, Instantaneous)"/1
  I_s/1 -> "Power (3ph, Instantaneous)"/2

== system Neutral_current_Load_balancing/PWM signal Generation/Hysteresis current controller ==
  In1 : Inport
  In2 : Inport  Port=2
  In3 : Inport  Port=3
  Hysteresis Current Controller (Three-Phase) : eeHysteresisControl/Hysteresis Current Controller (Three-Phase)  h=1  Ts=-1
      settings: SourceProductName=Simscape Electrical  SourceProductBaseCode=PS
  Mux : Mux  Inputs=3
  Out1 : Outport
  wires:
  In1/1 -> Mux/1
  Mux/1 -> Hysteresis Current Controller (Three-Phase)/1
  In2/1 -> Mux/2
  Hysteresis Current Controller (Three-Phase)/1 -> Out1/1
  [Ir] -> Hysteresis Current Controller (Three-Phase)/2
  In3/1 -> Mux/3

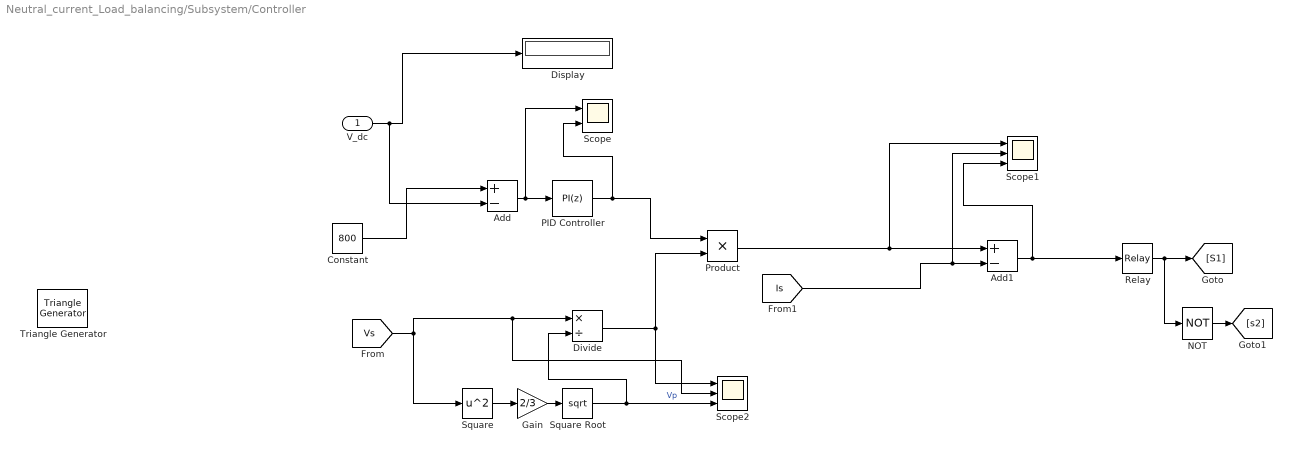
== system Neutral_current_Load_balancing/Subsystem/Controller ==
  V_dc : Inport
  Add : Sum  Inputs=+-
  Add1 : Sum  Inputs=+-
  Constant : Constant  Value=800
  Display : Display
  Divide : Product  Inputs=*/
  Gain : Gain  Gain=2/3
  NOT : Logic  Operator=NOT  IconShape=distinctive  AllPortsSameDT=off  OutDataTypeStr=boolean
  PID Controller : simulink/Continuous/PID Controller  Controller=PI  Form=Parallel  TimeDomain=Discrete-time  SampleTime=1e-6  IntegratorMethod=Forward Euler  FilterMethod=Forward Euler  ControllerParametersSource=internal  P=0.1  I=0.8  D=0  UseFilter=on  N=100  TunerSelectOption=Transfer Function Based (PID Tuner App)  InitialConditionSource=internal  InitialConditionForIntegrator=0  InitialConditionForFilter=0  DifferentiatorICPrevScaledInput=0  ExternalReset=none  TrackingMode=off  Kt=1  LimitOutput=off  UpperSaturationLimit=50  LowerSaturationLimit=-50  LinearizeAsGain=on  AntiWindupMode=none  Kb=1  POutMin=[]  POutMax=[]  IOutMin=[]  IOutMax=[]  DOutMin=[]  DOutMax=[]  NOutMin=[]  NOutMax=[]  SumOutMin=[]  SumOutMax=[]  SaturationOutMin=[]  SaturationOutMax=[]  PParamMin=[]  PParamMax=[]  IParamMin=[]  IParamMax=[]  DParamMin=[]  DParamMax=[]  NParamMin=[]  NParamMax=[]  KbParamMin=[]  KbParamMax=[]  KtParamMin=[]  KtParamMax=[]  KbOutMin=[]  KbOutMax=[]  KtOutMin=[]  KtOutMax=[]  IntegratorOutMin=[]  IntegratorOutMax=[]  FilterOutMin=[]  FilterOutMax=[]  SumI1OutMin=[]  SumI1OutMax=[]  SumI2OutMin=[]  SumI2OutMax=[]  SumI3OutMin=[]  SumI3OutMax=[]  SumI4OutMin=[]  SumI4OutMax=[]  SumDOutMin=[]  SumDOutMax=[]  DifferentiatorOutMin=[]  DifferentiatorOutMax=[]  FilterDiffOutCoefMin=[]  FilterDiffOutCoefMax=[]  ReciprocalOutMin=[]  ReciprocalOutMax=[]  SumDenOutMin=[]  SumDenOutMax=[]  SumNumOutMin=[]  SumNumOutMax=[]  DivideOutMin=[]  DivideOutMax=[]  IntegratorContinuousStateAttributes=''  IntegratorStateMustResolveToSignalObject=off  IntegratorRTWStateStorageClass=Auto  FilterContinuousStateAttributes=''  FilterStateMustResolveToSignalObject=off  FilterRTWStateStorageClass=Auto  ParallelPVariant=InternalParameters  IdealPVariant=Disabled  IVariant=InternalParameters  DVariant=Disabled  IntegratorVariant=Discrete  SatVariant=Disabled  AWVariant=Passthrough  PCopyVariant=Disabled  TRVariant=Disabled  FdbkBlocksVariant=Forward  IdealPFdbkVariant=Disabled  SatFdbkVariant=Disabled  DerivativeFilterVariant=Disabled  NVariant=Disabled  NCopyVariant=Disabled_SignalSpec  FilterICVariant=Disabled  IntegratorICVariant=InternalICs  ExternalResetVariant=Disabled  TRSumVariant=Passthrough  SumFdbkVariant=Disabled  SumVariant=Sum_PI
  Product : Product
  Relay : Relay  OnSwitchValue=1  OffSwitchValue=-1
  Scope : Scope  NumInputPorts=2
  Scope1 : Scope  NumInputPorts=3
  Scope2 : Scope  NumInputPorts=3
  Square : Math  Operator=square  SignedPower=off  SaturateOnIntegerOverflow=on
  Square Root : Sqrt  SaturateOnIntegerOverflow=on
  Triangle Generator : powerlib_meascontrol/Pulse & Signal Generators/Triangle Generator  Freq=1e3  Phase=90  Ts=0
      settings: SourceProductName=Simscape Electrical
  wires:
  V_dc/1 -> Display/1, Add/2
  Add/1 -> Scope/1, PID Controller/1
  [Vs] -> Square/1, Scope2/2, Divide/1
  PID Controller/1 -> Scope/2, Product/1
  Divide/1 -> Product/2, Scope2/1
  Product/1 -> Scope1/1, Add1/1
  Add1/1 -> Scope1/3, Relay/1
  [Is] -> Scope1/2, Add1/2
  Relay/1 -> NOT/1, [S1]
  NOT/1 -> [s2]
  Constant/1 -> Add/1
  Square/1 -> Gain/1
  Gain/1 -> Square Root/1
  Square Root/1 -> Scope2/3, Divide/2  "Vp"

== matlab function Neutral_current_Load_balancing/Subsystem1/MATLAB Function ==
  data: vsa input; isa_star output; vsb input; vsc input; idls input; isb_star output; isc_star output; usa output; usb output; usc output; vp output
function [isa_star , isb_star ,isc_star,usa,usb,usc,vp] = fcn(vsa,vsb,vsc,idls)

vp = sqrt((2/3)*(vsa^2+vsb^2+vsc^2));

usa = vsa/vp;

usb = vsb / vp;

usc = vsc /vp;

isa_star = usa*idls;

isb_star = usb * idls;

isc_star = usc*idls;
